simulink subsystem "rss_FaltResp"  (R2023a)
settings: Solver=VariableStepAuto  StartTime=0.0  StopTime=10.0  RelTol=1e-3
undefined symbols (not defined in the file): Cdbl_numFaltDiaNum, ENM_SYS_STATUS, Gbol_enLmpHmeStop_C, Gs16_nLmpHmeRefMechSpd_C, Gs16_nMaxRefMechSpd_C, Gs16_nMotoTmpStallRefMechSpd_C, Gs16_trqTmpStallTqUpLim_C, Gs16_trqTqUpLim_C, Gu16_ctLmpHmeDurCnt_C, Gu16_uLimHmeSplyVltgConfTrs_C, Gu16_uLimHmeSplyVltgRcvyTrs_C
libraries: simulink x5, vhit_control_library x1
settings Model: Creator=xiaoqiang.yuan  LastModifiedBy=xiaoqiang.yuan

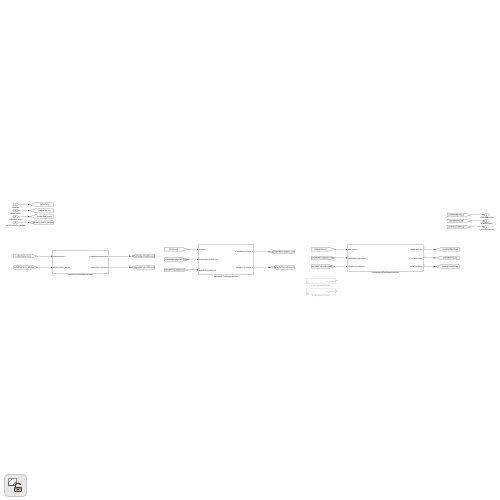
[thumbnail: Simulink's stored preview of the top-level diagram]
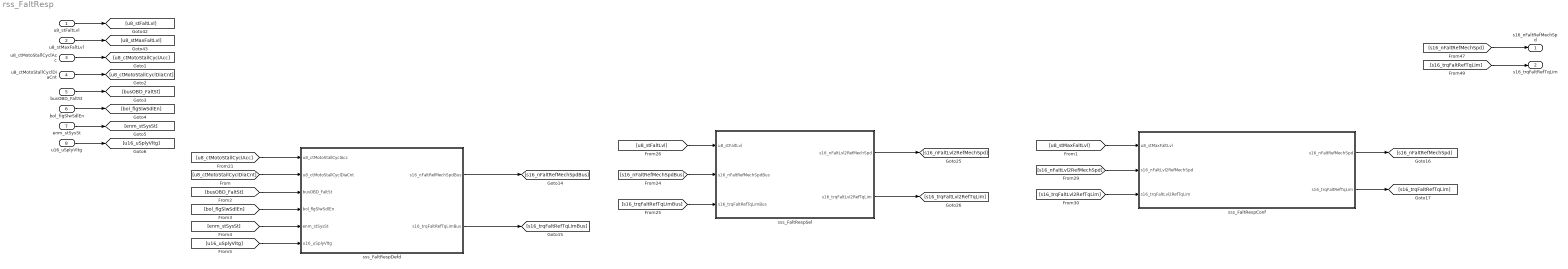
== system rss_FaltResp ==
  u8_stFaltLvl : Inport  OutDataTypeStr=uint8
  u8_stMaxFaltLvl : Inport  Port=2  OutDataTypeStr=uint8
  u8_ctMotoStallCyclAcc : Inport  Port=3  OutDataTypeStr=uint8
  u8_ctMotoStallCyclDiaCnt : Inport  Port=4  OutDataTypeStr=uint8
  busOBD_FaltSt : Inport  Port=5  OutDataTypeStr=Bus: BUS_OBD_FALT_STS
  bol_flgSlwSdlEn : Inport  Port=6  OutDataTypeStr=boolean
  enm_stSysSt : Inport  Port=7  OutDataTypeStr=Enum: ENM_SYS_STATUS
  u16_uSplyVltg : Inport  Port=8
  sss_FaltRespConf : Subsystem
  sss_FaltRespDefd : Subsystem
  sss_FaltRespSel : Subsystem
  s16_nFaltRefMechSpd : Outport  OutDataTypeStr=dt_Standardize_s16p15b0
  s16_trqFaltRefTqLim : Outport  Port=2  OutDataTypeStr=dt_Standardize_s16p15b0
  wires:
  u8_stFaltLvl/1 -> [u8_stFaltLvl]
  u8_stMaxFaltLvl/1 -> [u8_stMaxFaltLvl]
  u8_ctMotoStallCyclAcc/1 -> [u8_ctMotoStallCyclAcc]
  [u8_ctMotoStallCyclAcc] -> sss_FaltRespDefd/1(u8_ctMotoStallCyclAcc)
  sss_FaltRespDefd/1(s16_nFaltRefMechSpdBus) -> [s16_nFaltRefMechSpdBus]
  sss_FaltRespDefd/2(s16_trqFaltRefTqLimBus) -> [s16_trqFaltRefTqLimBus]
  [s16_trqFaltRefTqLimBus] -> sss_FaltRespSel/3(s16_trqFaltRefTqLimBus)
  [s16_nFaltRefMechSpdBus] -> sss_FaltRespSel/2(s16_nFaltRefMechSpdBus)
  [u8_stFaltLvl] -> sss_FaltRespSel/1(u8_stFaltLvl)
  sss_FaltRespSel/2(s16_trqFaltLvl2RefTqLim) -> [s16_trqFaltLvl2RefTqLim]
  sss_FaltRespSel/1(s16_nFaltLvl2RefMechSpd) -> [s16_nFaltLvl2RefMechSpd]
  sss_FaltRespConf/1(s16_nFaltRefMechSpd) -> [s16_nFaltRefMechSpd]
  sss_FaltRespConf/2(s16_trqFaltRefTqLim) -> [s16_trqFaltRefTqLim]
  [s16_nFaltRefMechSpd] -> s16_nFaltRefMechSpd/1
  [s16_trqFaltRefTqLim] -> s16_trqFaltRefTqLim/1
  [u8_stMaxFaltLvl] -> sss_FaltRespConf/1(u8_stMaxFaltLvl)
  u8_ctMotoStallCyclDiaCnt/1 -> [u8_ctMotoStallCyclDiaCnt]
  [u8_ctMotoStallCyclDiaCnt] -> sss_FaltRespDefd/2(u8_ctMotoStallCyclDiaCnt)
  busOBD_FaltSt/1 -> [busOBD_FaltSt]
  [busOBD_FaltSt] -> sss_FaltRespDefd/3(busOBD_FaltSt)
  bol_flgSlwSdlEn/1 -> [bol_flgSlwSdlEn]
  [bol_flgSlwSdlEn] -> sss_FaltRespDefd/4(bol_flgSlwSdlEn)
  enm_stSysSt/1 -> [enm_stSysSt]
  [enm_stSysSt] -> sss_FaltRespDefd/5(enm_stSysSt)
  [s16_nFaltLvl2RefMechSpd] -> sss_FaltRespConf/2(s16_nFaltLvl2RefMechSpd)
  [s16_trqFaltLvl2RefTqLim] -> sss_FaltRespConf/3(s16_trqFaltLvl2RefTqLim)
  u16_uSplyVltg/1 -> [u16_uSplyVltg]
  [u16_uSplyVltg] -> sss_FaltRespDefd/6(u16_uSplyVltg)

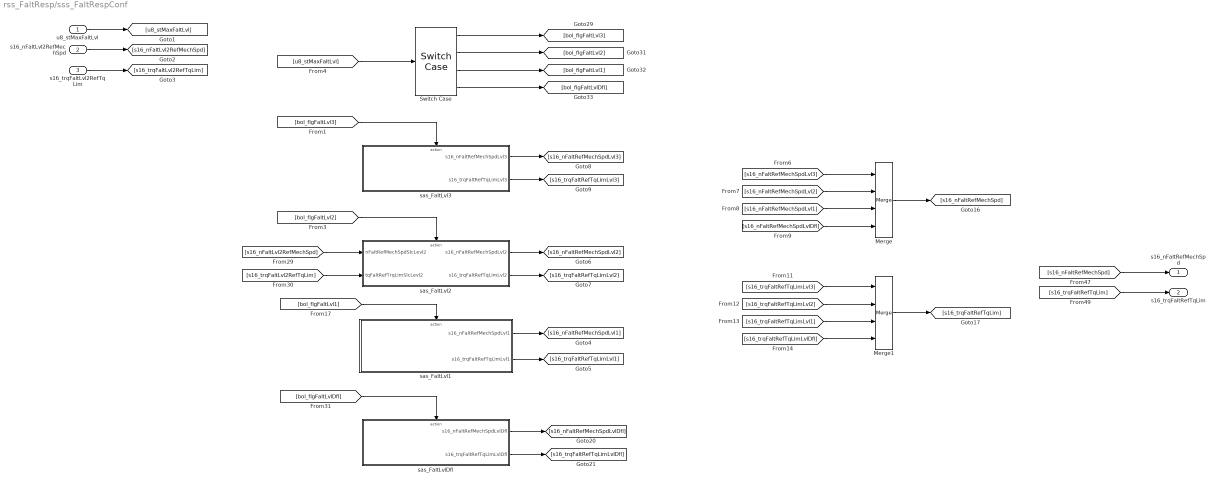
== system rss_FaltResp/sss_FaltRespConf ==
  u8_stMaxFaltLvl : Inport
  s16_nFaltLvl2RefMechSpd : Inport  Port=2
  s16_trqFaltLvl2RefTqLim : Inport  Port=3
  Merge : Merge  Inputs=4
  Merge1 : Merge  Inputs=4
  Switch Case : SwitchCase  CaseConditions={3,2,1}
  sas_FaltLvl1 : Subsystem  TreatAsAtomicUnit=on
  sas_FaltLvl2 : Subsystem  TreatAsAtomicUnit=on
  sas_FaltLvl3 : Subsystem  TreatAsAtomicUnit=on
  sas_FaltLvlDfl : Subsystem  TreatAsAtomicUnit=on
  s16_nFaltRefMechSpd : Outport
  s16_trqFaltRefTqLim : Outport  Port=2
  wires:
  [s16_trqFaltRefTqLimLvlDfl] -> Merge1/4
  [s16_trqFaltRefTqLimLvl1] -> Merge1/3
  [s16_trqFaltRefTqLimLvl2] -> Merge1/2
  [s16_trqFaltRefTqLimLvl3] -> Merge1/1
  [s16_nFaltRefMechSpdLvlDfl] -> Merge/4
  [s16_nFaltRefMechSpdLvl1] -> Merge/3
  [s16_nFaltRefMechSpdLvl2] -> Merge/2
  [s16_nFaltRefMechSpdLvl3] -> Merge/1
  Switch Case/2 -> [bol_flgFaltLvl2]
  s16_trqFaltLvl2RefTqLim/1 -> [s16_trqFaltLvl2RefTqLim]
  s16_nFaltLvl2RefMechSpd/1 -> [s16_nFaltLvl2RefMechSpd]
  u8_stMaxFaltLvl/1 -> [u8_stMaxFaltLvl]
  sas_FaltLvl1/1(s16_nFaltRefMechSpdLvl1) -> [s16_nFaltRefMechSpdLvl1]
  sas_FaltLvl1/2(s16_trqFaltRefTqLimLvl1) -> [s16_trqFaltRefTqLimLvl1]
  sas_FaltLvlDfl/1(s16_nFaltRefMechSpdLvlDfl) -> [s16_nFaltRefMechSpdLvlDfl]
  Merge/1 -> [s16_nFaltRefMechSpd]
  [s16_nFaltLvl2RefMechSpd] -> sas_FaltLvl2/1(nFaltRefMechSpdSlcLevl2)
  sas_FaltLvl3/1(s16_nFaltRefMechSpdLvl3) -> [s16_nFaltRefMechSpdLvl3]
  [bol_flgFaltLvlDfl] -> sas_FaltLvlDfl/Action
  sas_FaltLvl3/2(s16_trqFaltRefTqLimLvl3) -> [s16_trqFaltRefTqLimLvl3]
  sas_FaltLvlDfl/2(s16_trqFaltRefTqLimLvlDfl) -> [s16_trqFaltRefTqLimLvlDfl]
  [bol_flgFaltLvl2] -> sas_FaltLvl2/Action
  Switch Case/4 -> [bol_flgFaltLvlDfl]
  Merge1/1 -> [s16_trqFaltRefTqLim]
  Switch Case/3 -> [bol_flgFaltLvl1]
  [u8_stMaxFaltLvl] -> Switch Case/1
  [s16_trqFaltRefTqLim] -> s16_trqFaltRefTqLim/1
  [bol_flgFaltLvl3] -> sas_FaltLvl3/Action
  sas_FaltLvl2/2(s16_trqFaltRefTqLimLvl2) -> [s16_trqFaltRefTqLimLvl2]
  sas_FaltLvl2/1(s16_nFaltRefMechSpdLvl2) -> [s16_nFaltRefMechSpdLvl2]
  [bol_flgFaltLvl1] -> sas_FaltLvl1/Action
  Switch Case/1 -> [bol_flgFaltLvl3]
  [s16_trqFaltLvl2RefTqLim] -> sas_FaltLvl2/2(tqFaltRefTrqLimSlcLevl2)
  [s16_nFaltRefMechSpd] -> s16_nFaltRefMechSpd/1

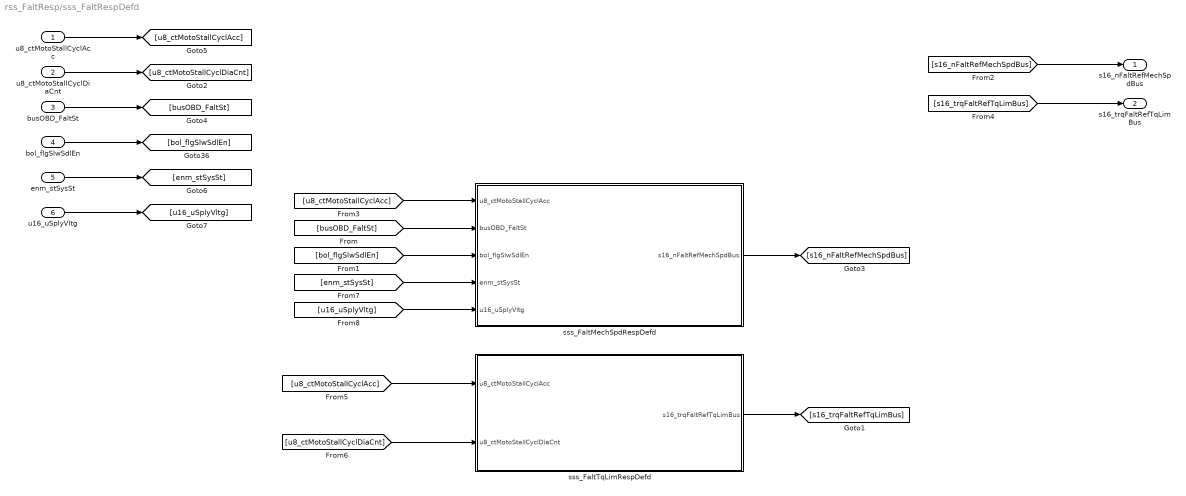
== system rss_FaltResp/sss_FaltRespDefd ==
  u8_ctMotoStallCyclAcc : Inport
  u8_ctMotoStallCyclDiaCnt : Inport  Port=2
  busOBD_FaltSt : Inport  Port=3
  bol_flgSlwSdlEn : Inport  Port=4
  enm_stSysSt : Inport  Port=5
  u16_uSplyVltg : Inport  Port=6
  sss_FaltMechSpdRespDefd : Subsystem
  sss_FaltTqLimRespDefd : Subsystem
  s16_nFaltRefMechSpdBus : Outport
  s16_trqFaltRefTqLimBus : Outport  Port=2
  wires:
  [u16_uSplyVltg] -> sss_FaltMechSpdRespDefd/5(u16_uSplyVltg)
  u16_uSplyVltg/1 -> [u16_uSplyVltg]
  [enm_stSysSt] -> sss_FaltMechSpdRespDefd/4(enm_stSysSt)
  enm_stSysSt/1 -> [enm_stSysSt]
  [bol_flgSlwSdlEn] -> sss_FaltMechSpdRespDefd/3(bol_flgSlwSdlEn)
  bol_flgSlwSdlEn/1 -> [bol_flgSlwSdlEn]
  [busOBD_FaltSt] -> sss_FaltMechSpdRespDefd/2(busOBD_FaltSt)
  busOBD_FaltSt/1 -> [busOBD_FaltSt]
  [u8_ctMotoStallCyclAcc] -> sss_FaltMechSpdRespDefd/1(u8_ctMotoStallCyclAcc)
  sss_FaltTqLimRespDefd/1(s16_trqFaltRefTqLimBus) -> [s16_trqFaltRefTqLimBus]
  sss_FaltMechSpdRespDefd/1(s16_nFaltRefMechSpdBus) -> [s16_nFaltRefMechSpdBus]
  [u8_ctMotoStallCyclDiaCnt] -> sss_FaltTqLimRespDefd/2(u8_ctMotoStallCyclDiaCnt)
  [u8_ctMotoStallCyclAcc] -> sss_FaltTqLimRespDefd/1(u8_ctMotoStallCyclAcc)
  u8_ctMotoStallCyclDiaCnt/1 -> [u8_ctMotoStallCyclDiaCnt]
  u8_ctMotoStallCyclAcc/1 -> [u8_ctMotoStallCyclAcc]
  [s16_trqFaltRefTqLimBus] -> s16_trqFaltRefTqLimBus/1
  [s16_nFaltRefMechSpdBus] -> s16_nFaltRefMechSpdBus/1

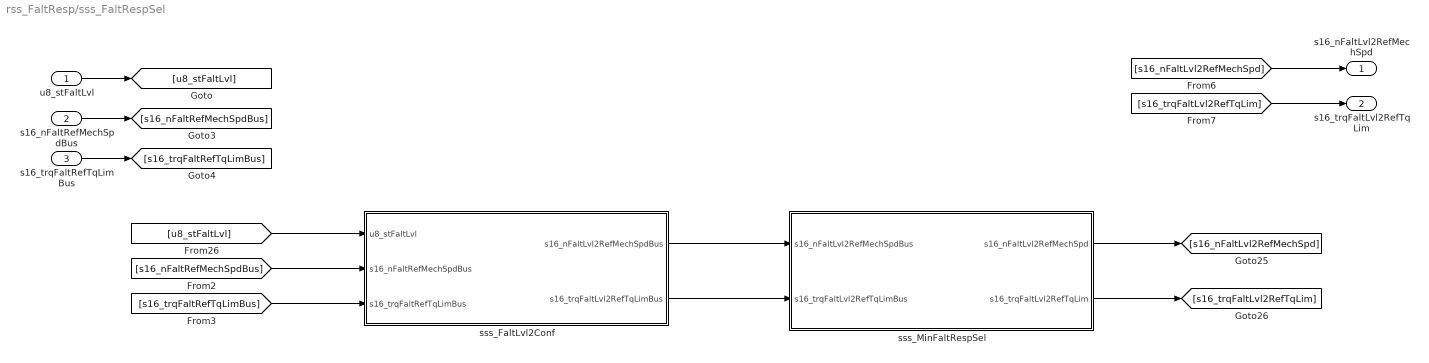
== system rss_FaltResp/sss_FaltRespSel ==
  u8_stFaltLvl : Inport
  s16_nFaltRefMechSpdBus : Inport  Port=2
  s16_trqFaltRefTqLimBus : Inport  Port=3
  sss_FaltLvl2Conf : Subsystem  TreatAsAtomicUnit=on
      settings: RTWSystemCode=Nonreusable function
  sss_MinFaltRespSel : Subsystem
      settings: RTWSystemCode=Nonreusable function
  s16_nFaltLvl2RefMechSpd : Outport
  s16_trqFaltLvl2RefTqLim : Outport  Port=2
  wires:
  sss_FaltLvl2Conf/2(s16_trqFaltLvl2RefTqLimBus) -> sss_MinFaltRespSel/2(s16_trqFaltLvl2RefTqLimBus)
  sss_FaltLvl2Conf/1(s16_nFaltLvl2RefMechSpdBus) -> sss_MinFaltRespSel/1(s16_nFaltLvl2RefMechSpdBus)
  sss_MinFaltRespSel/2(s16_trqFaltLvl2RefTqLim) -> [s16_trqFaltLvl2RefTqLim]
  sss_MinFaltRespSel/1(s16_nFaltLvl2RefMechSpd) -> [s16_nFaltLvl2RefMechSpd]
  [s16_trqFaltLvl2RefTqLim] -> s16_trqFaltLvl2RefTqLim/1
  [s16_nFaltLvl2RefMechSpd] -> s16_nFaltLvl2RefMechSpd/1
  [s16_trqFaltRefTqLimBus] -> sss_FaltLvl2Conf/3(s16_trqFaltRefTqLimBus)
  [s16_nFaltRefMechSpdBus] -> sss_FaltLvl2Conf/2(s16_nFaltRefMechSpdBus)
  [u8_stFaltLvl] -> sss_FaltLvl2Conf/1(u8_stFaltLvl)
  s16_nFaltRefMechSpdBus/1 -> [s16_nFaltRefMechSpdBus]
  s16_trqFaltRefTqLimBus/1 -> [s16_trqFaltRefTqLimBus]
  u8_stFaltLvl/1 -> [u8_stFaltLvl]

== system rss_FaltResp/sss_FaltRespConf/sas_FaltLvl1 ==
  Action Port : ActionPort
  Constant : Constant  Value=Gs16_nMaxRefMechSpd_C
  Constant1 : Constant  Value=Gs16_trqTqUpLim_C
  s16_nFaltRefMechSpdLvl1 : Outport
  s16_trqFaltRefTqLimLvl1 : Outport  Port=2
  wires:
  Constant/1 -> s16_nFaltRefMechSpdLvl1/1
  Constant1/1 -> s16_trqFaltRefTqLimLvl1/1

== system rss_FaltResp/sss_FaltRespConf/sas_FaltLvl2 ==
  nFaltRefMechSpdSlcLevl2 : Inport
  tqFaltRefTrqLimSlcLevl2 : Inport  Port=2
  Action Port : ActionPort
  s16_nFaltRefMechSpdLvl2 : Outport
  s16_trqFaltRefTqLimLvl2 : Outport  Port=2
  wires:
  nFaltRefMechSpdSlcLevl2/1 -> s16_nFaltRefMechSpdLvl2/1
  tqFaltRefTrqLimSlcLevl2/1 -> s16_trqFaltRefTqLimLvl2/1

== system rss_FaltResp/sss_FaltRespConf/sas_FaltLvl3 ==
  Action Port : ActionPort
  Constant : Constant  Value=0  OutDataTypeStr=dt_Standardize_s16p15b0
  Constant1 : Constant  Value=0  OutDataTypeStr=dt_Standardize_s16p15b0
  s16_nFaltRefMechSpdLvl3 : Outport
  s16_trqFaltRefTqLimLvl3 : Outport  Port=2
  wires:
  Constant/1 -> s16_nFaltRefMechSpdLvl3/1
  Constant1/1 -> s16_trqFaltRefTqLimLvl3/1

== system rss_FaltResp/sss_FaltRespConf/sas_FaltLvlDfl ==
  Action Port : ActionPort
  Constant : Constant  Value=Gs16_nMaxRefMechSpd_C
  Constant1 : Constant  Value=Gs16_trqTqUpLim_C
  s16_nFaltRefMechSpdLvlDfl : Outport
  s16_trqFaltRefTqLimLvlDfl : Outport  Port=2
  wires:
  Constant/1 -> s16_nFaltRefMechSpdLvlDfl/1
  Constant1/1 -> s16_trqFaltRefTqLimLvlDfl/1

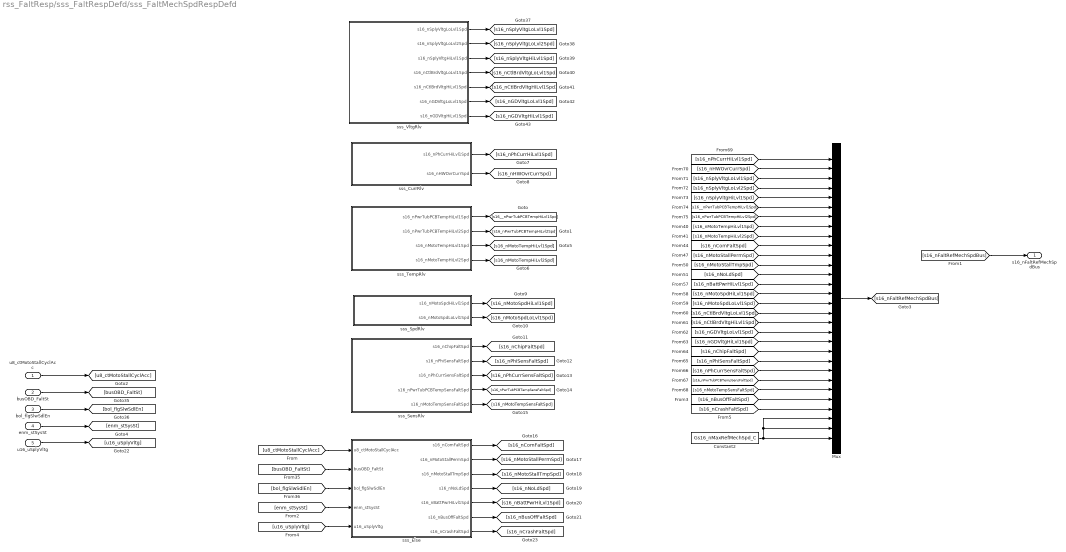
== system rss_FaltResp/sss_FaltRespDefd/sss_FaltMechSpdRespDefd ==
  u8_ctMotoStallCyclAcc : Inport
  busOBD_FaltSt : Inport  Port=2
  bol_flgSlwSdlEn : Inport  Port=3
  enm_stSysSt : Inport  Port=4
  u16_uSplyVltg : Inport  Port=5
  Constant2 : Constant  Value=Gs16_nMaxRefMechSpd_C
  Mux : Mux  Inputs=30
  sss_CurrRlv : Subsystem
  sss_Else : Subsystem
  sss_SensRlv : Subsystem
  sss_SpdRlv : Subsystem
  sss_TempRlv : Subsystem
  sss_VltgRlv : Subsystem
  s16_nFaltRefMechSpdBus : Outport
  wires:
  [s16_nCrashFaltSpd] -> Mux/27
  sss_Else/7(s16_nCrashFaltSpd) -> [s16_nCrashFaltSpd]
  [u16_uSplyVltg] -> sss_Else/5(u16_uSplyVltg)
  u16_uSplyVltg/1 -> [u16_uSplyVltg]
  [s16_nBusOffFaltSpd] -> Mux/26
  sss_Else/6(s16_nBusOffFaltSpd) -> [s16_nBusOffFaltSpd]
  [enm_stSysSt] -> sss_Else/4(enm_stSysSt)
  enm_stSysSt/1 -> [enm_stSysSt]
  [u8_ctMotoStallCyclAcc] -> sss_Else/1(u8_ctMotoStallCyclAcc)
  [bol_flgSlwSdlEn] -> sss_Else/3(bol_flgSlwSdlEn)
  [busOBD_FaltSt] -> sss_Else/2(busOBD_FaltSt)
  sss_Else/1(s16_nComFaltSpd) -> [s16_nComFaltSpd]
  sss_Else/2(s16_nMotoStallPermSpd) -> [s16_nMotoStallPermSpd]
  sss_Else/3(s16_nMotoStallTmpSpd) -> [s16_nMotoStallTmpSpd]
  sss_Else/4(s16_nNoLdSpd) -> [s16_nNoLdSpd]
  sss_Else/5(s16_nBattPwrHiLvl1Spd) -> [s16_nBattPwrHiLvl1Spd]
  sss_SensRlv/5(s16_nMotoTempSensFaltSpd) -> [s16_nMotoTempSensFaltSpd]
  sss_SensRlv/4(s16_nPwrTubPCBTempSensFaltSpd) -> [s16_nPwrTubPCBTempSensFaltSpd]
  sss_SensRlv/3(s16_nPhCurrSensFaltSpd) -> [s16_nPhCurrSensFaltSpd]
  sss_SensRlv/2(s16_nPhiSensFaltSpd) -> [s16_nPhiSensFaltSpd]
  sss_SensRlv/1(s16_nChipFaltSpd) -> [s16_nChipFaltSpd]
  sss_SpdRlv/2(s16_nMotoSpdLoLvl1Spd) -> [s16_nMotoSpdLoLvl1Spd]
  sss_SpdRlv/1(s16_nMotoSpdHiLvl1Spd) -> [s16_nMotoSpdHiLvl1Spd]
  sss_TempRlv/4(s16_nMotoTempHiLvl2Spd) -> [s16_nMotoTempHiLvl2Spd]
  sss_TempRlv/3(s16_nMotoTempHiLvl1Spd) -> [s16_nMotoTempHiLvl1Spd]
  sss_TempRlv/2(s16_nPwrTubPCBTempHiLvl2Spd) -> [s16_nPwrTubPCBTempHiLvl2Spd]
  sss_TempRlv/1(s16_nPwrTubPCBTempHiLvl1Spd) -> [s16__nPwrTubPCBTempHiLvl1Spd]
  sss_CurrRlv/2(s16_nHWOvrCurrSpd) -> [s16_nHWOvrCurrSpd]
  sss_CurrRlv/1(s16_nPhCurrHiLvl1Spd) -> [s16_nPhCurrHiLvl1Spd]
  Mux/1 -> [s16_nFaltRefMechSpdBus]
  [s16_nPhCurrSensFaltSpd] -> Mux/23
  [s16_nMotoStallTmpSpd] -> Mux/12
  Constant2/1 -> Mux/30, Mux/29, Mux/28
  [s16_nSplyVltgHiLvl1Spd] -> Mux/5
  [s16_nSplyVltgLoLvl1Spd] -> Mux/3
  [s16__nPwrTubPCBTempHiLvl1Spd] -> Mux/6
  [s16_nGDVltgLoLvl1Spd] -> Mux/19
  [s16_nHWOvrCurrSpd] -> Mux/2
  [s16_nMotoSpdHiLvl1Spd] -> Mux/15
  [s16_nPwrTubPCBTempSensFaltSpd] -> Mux/24
  [s16_nNoLdSpd] -> Mux/13
  [s16_nChipFaltSpd] -> Mux/21
  [s16_nMotoTempSensFaltSpd] -> Mux/25
  [s16_nPhCurrHiLvl1Spd] -> Mux/1
  [s16_nCtlBrdVltgLoLvl1Spd] -> Mux/17
  [s16_nPhiSensFaltSpd] -> Mux/22
  [s16_nGDVltgHiLvl1Spd] -> Mux/20
  [s16_nCtlBrdVltgHiLvl1Spd] -> Mux/18
  [s16_nComFaltSpd] -> Mux/10
  [s16_nMotoSpdLoLvl1Spd] -> Mux/16
  [s16_nMotoStallPermSpd] -> Mux/11
  [s16_nBattPwrHiLvl1Spd] -> Mux/14
  [s16_nPwrTubPCBTempHiLvl2Spd] -> Mux/7
  [s16_nMotoTempHiLvl1Spd] -> Mux/8
  [s16_nMotoTempHiLvl2Spd] -> Mux/9
  [s16_nSplyVltgLoLvl2Spd] -> Mux/4
  bol_flgSlwSdlEn/1 -> [bol_flgSlwSdlEn]
  busOBD_FaltSt/1 -> [busOBD_FaltSt]
  [s16_nFaltRefMechSpdBus] -> s16_nFaltRefMechSpdBus/1
  u8_ctMotoStallCyclAcc/1 -> [u8_ctMotoStallCyclAcc]
  sss_VltgRlv/5(s16_nCtlBrdVltgHiLvl1Spd) -> [s16_nCtlBrdVltgHiLvl1Spd]
  sss_VltgRlv/6(s16_nGDVltgLoLvl1Spd) -> [s16_nGDVltgLoLvl1Spd]
  sss_VltgRlv/2(s16_nSplyVltgLoLvl2Spd) -> [s16_nSplyVltgLoLvl2Spd]
  sss_VltgRlv/3(s16_nSplyVltgHiLvl1Spd) -> [s16_nSplyVltgHiLvl1Spd]
  sss_VltgRlv/7(s16_nGDVltgHiLvl1Spd) -> [s16_nGDVltgHiLvl1Spd]
  sss_VltgRlv/4(s16_nCtlBrdVltgLoLvl1Spd) -> [s16_nCtlBrdVltgLoLvl1Spd]
  sss_VltgRlv/1(s16_nSplyVltgLoLvl1Spd) -> [s16_nSplyVltgLoLvl1Spd]

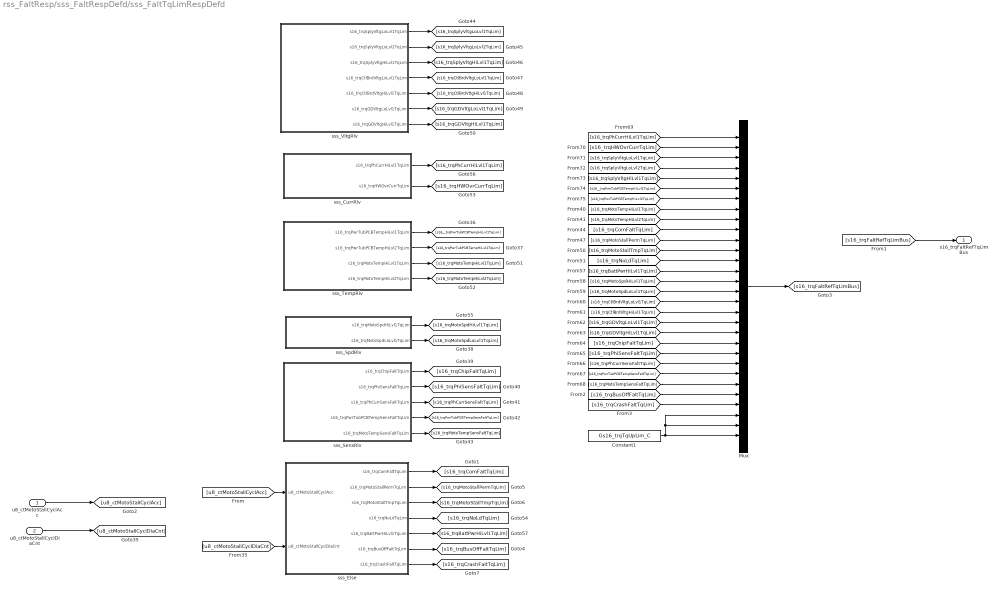
== system rss_FaltResp/sss_FaltRespDefd/sss_FaltTqLimRespDefd ==
  u8_ctMotoStallCyclAcc : Inport
  u8_ctMotoStallCyclDiaCnt : Inport  Port=2
  Constant1 : Constant  Value=Gs16_trqTqUpLim_C
  Mux : Mux  Inputs=30
  sss_CurrRlv : Subsystem
  sss_Else : Subsystem
  sss_SensRlv : Subsystem
  sss_SpdRlv : Subsystem
  sss_TempRlv : Subsystem
  sss_VltgRlv : Subsystem
  s16_trqFaltRefTqLimBus : Outport
  wires:
  [s16_trqCrashFaltTqLim] -> Mux/27
  sss_Else/7(s16_trqCrashFaltTqLim) -> [s16_trqCrashFaltTqLim]
  [s16_trqBusOffFaltTqLim] -> Mux/26
  sss_Else/6(s16_trqBusOffFaltTqLim) -> [s16_trqBusOffFaltTqLim]
  [u8_ctMotoStallCyclDiaCnt] -> sss_Else/2(u8_ctMotoStallCyclDiaCnt)
  [u8_ctMotoStallCyclAcc] -> sss_Else/1(u8_ctMotoStallCyclAcc)
  sss_Else/4(s16_trqNoLdTqLim) -> [s16_trqNoLdTqLim]
  sss_Else/3(s16_trqMotoStallTmpTqLim) -> [s16_trqMotoStallTmpTqLim]
  sss_Else/1(s16_trqComFaltTqLim) -> [s16_trqComFaltTqLim]
  sss_Else/2(s16_trqMotoStallPermTqLim) -> [s16_trqMotoStallPermTqLim]
  sss_Else/5(s16_trqBattPwrHiLvl1TqLim) -> [s16_trqBattPwrHiLvl1TqLim]
  sss_SensRlv/3(s16_trqPhCurrSensFaltTqLim) -> [s16_trqPhCurrSensFaltTqLim]
  sss_SpdRlv/1(s16_trqMotoSpdHiLvl1TqLim) -> [s16_trqMotoSpdHiLvl1TqLim]
  sss_TempRlv/3(s16_trqMotoTempHiLvl1TqLim) -> [s16_trqMotoTempHiLvl1TqLim]
  sss_TempRlv/1(s16_trqPwrTubPCBTempHiLvl1TqLim) -> [s16__trqPwrTubPCBTempHiLvl1TqLim]
  sss_VltgRlv/2(s16_trqSplyVltgLoLvl2TqLim) -> [s16_trqSplyVltgLoLvl2TqLim]
  sss_CurrRlv/2(s16_trqHWOvrCurrTqLim) -> [s16_trqHWOvrCurrTqLim]
  sss_SensRlv/1(s16_trqChipFaltTqLim) -> [s16_trqChipFaltTqLim]
  sss_SpdRlv/2(s16_trqMotoSpdLoLvl1TqLim) -> [s16_trqMotoSpdLoLvl1TqLim]
  sss_TempRlv/4(s16_trqMotoTempHiLvl2TqLim) -> [s16_trqMotoTempHiLvl2TqLim]
  sss_VltgRlv/6(s16_trqGDVltgLoLvl1TqLim) -> [s16_trqGDVltgLoLvl1TqLim]
  sss_VltgRlv/3(s16_trqSplyVltgHiLvl1TqLim) -> [s16_trqSplyVltgHiLvl1TqLim]
  sss_SensRlv/2(s16_trqPhiSensFaltTqLim) -> [s16_trqPhiSensFaltTqLim]
  sss_SensRlv/4(s16_trqPwrTubPCBTempSensFaltTqLim) -> [s16_trqPwrTubPCBTempSensFaltTqLim]
  sss_VltgRlv/5(s16_trqCtlBrdVltgHiLvl1TqLim) -> [s16_trqCtlBrdVltgHiLvl1TqLim]
  sss_SensRlv/5(s16_trqMotoTempSensFaltTqLim) -> [s16_trqMotoTempSensFaltTqLim]
  sss_TempRlv/2(s16_trqPwrTubPCBTempHiLvl2TqLim) -> [s16_trqPwrTubPCBTempHiLvl2TqLim]
  sss_CurrRlv/1(s16_trqPhCurrHiLvl1TqLim) -> [s16_trqPhCurrHiLvl1TqLim]
  sss_VltgRlv/1(s16_trqSplyVltgLoLvl1TqLim) -> [s16_trqSplyVltgLoLvl1TqLim]
  sss_VltgRlv/4(s16_trqCtlBrdVltgLoLvl1TqLim) -> [s16_trqCtlBrdVltgLoLvl1TqLim]
  sss_VltgRlv/7(s16_trqGDVltgHiLvl1TqLim) -> [s16_trqGDVltgHiLvl1TqLim]
  Mux/1 -> [s16_trqFaltRefTqLimBus]
  [s16_trqChipFaltTqLim] -> Mux/21
  [s16_trqMotoTempHiLvl1TqLim] -> Mux/8
  [s16_trqMotoStallTmpTqLim] -> Mux/12
  [s16_trqPwrTubPCBTempHiLvl2TqLim] -> Mux/7
  [s16_trqPhCurrSensFaltTqLim] -> Mux/23
  [s16_trqMotoTempHiLvl2TqLim] -> Mux/9
  [s16_trqSplyVltgLoLvl2TqLim] -> Mux/4
  [s16_trqMotoStallPermTqLim] -> Mux/11
  [s16_trqComFaltTqLim] -> Mux/10
  [s16_trqCtlBrdVltgLoLvl1TqLim] -> Mux/17
  [s16_trqBattPwrHiLvl1TqLim] -> Mux/14
  [s16_trqGDVltgHiLvl1TqLim] -> Mux/20
  [s16_trqPhCurrHiLvl1TqLim] -> Mux/1
  [s16_trqMotoTempSensFaltTqLim] -> Mux/25
  [s16_trqCtlBrdVltgHiLvl1TqLim] -> Mux/18
  [s16_trqPhiSensFaltTqLim] -> Mux/22
  [s16_trqMotoSpdLoLvl1TqLim] -> Mux/16
  [s16__trqPwrTubPCBTempHiLvl1TqLim] -> Mux/6
  [s16_trqHWOvrCurrTqLim] -> Mux/2
  [s16_trqNoLdTqLim] -> Mux/13
  [s16_trqGDVltgLoLvl1TqLim] -> Mux/19
  [s16_trqMotoSpdHiLvl1TqLim] -> Mux/15
  [s16_trqSplyVltgLoLvl1TqLim] -> Mux/3
  [s16_trqSplyVltgHiLvl1TqLim] -> Mux/5
  [s16_trqPwrTubPCBTempSensFaltTqLim] -> Mux/24
  Constant1/1 -> Mux/30, Mux/29, Mux/28
  u8_ctMotoStallCyclDiaCnt/1 -> [u8_ctMotoStallCyclDiaCnt]
  u8_ctMotoStallCyclAcc/1 -> [u8_ctMotoStallCyclAcc]
  [s16_trqFaltRefTqLimBus] -> s16_trqFaltRefTqLimBus/1

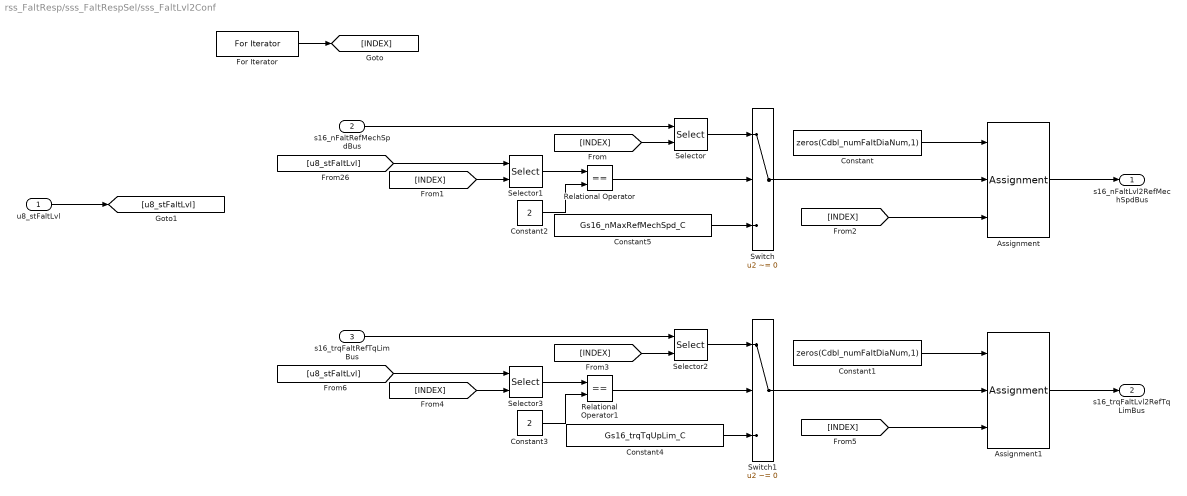
== system rss_FaltResp/sss_FaltRespSel/sss_FaltLvl2Conf ==
  u8_stFaltLvl : Inport
  s16_nFaltRefMechSpdBus : Inport  Port=2
  s16_trqFaltRefTqLimBus : Inport  Port=3
  Assignment : Assignment  DiagnosticForDimensions=Warning  IndexOptions=Index vector (port)  Indices=1  OutputSizes=1
  Assignment1 : Assignment  DiagnosticForDimensions=Warning  IndexOptions=Index vector (port)  Indices=1  OutputSizes=1
  Constant : Constant  Value=zeros(Cdbl_numFaltDiaNum,1)  OutDataTypeStr=dt_Standardize_s16p15b0
  Constant1 : Constant  Value=zeros(Cdbl_numFaltDiaNum,1)  OutDataTypeStr=dt_Standardize_s16p15b0
  Constant2 : Constant  Value=2  OutDataTypeStr=uint8
  Constant3 : Constant  Value=2  OutDataTypeStr=uint8
  Constant4 : Constant  Value=Gs16_trqTqUpLim_C
  Constant5 : Constant  Value=Gs16_nMaxRefMechSpd_C
  For Iterator : ForIterator  IterationLimit=Cdbl_numFaltDiaNum  IterationVariableDataType=uint8
  Relational Operator : RelationalOperator  Operator===  OutDataTypeStr=boolean  RndMeth=Simplest  InputSameDT=off
  Relational Operator1 : RelationalOperator  Operator===  OutDataTypeStr=boolean  RndMeth=Simplest  InputSameDT=off
  Selector{,1..3} (4 alike) : Selector  InputPortWidth=Cdbl_numFaltDiaNum  IndexOptions=Index vector (port)  Indices=[1 3]  OutputSizes=1
  Switch : Switch  Criteria=u2 ~= 0  SaturateOnIntegerOverflow=off  InputSameDT=off
  Switch1 : Switch  Criteria=u2 ~= 0  SaturateOnIntegerOverflow=off  InputSameDT=off
  s16_nFaltLvl2RefMechSpdBus : Outport
  s16_trqFaltLvl2RefTqLimBus : Outport  Port=2
  wires:
  [INDEX] -> Assignment/3
  Constant/1 -> Assignment/1
  Switch/1 -> Assignment/2
  [INDEX] -> Selector1/2
  [INDEX] -> Selector/2
  For Iterator/1 -> [INDEX]
  s16_nFaltRefMechSpdBus/1 -> Selector/1
  Constant5/1 -> Switch/3
  Selector/1 -> Switch/1
  Selector1/1 -> Relational Operator/1
  Constant2/1 -> Relational Operator/2
  Relational Operator/1 -> Switch/2
  Assignment/1 -> s16_nFaltLvl2RefMechSpdBus/1
  u8_stFaltLvl/1 -> [u8_stFaltLvl]
  [u8_stFaltLvl] -> Selector1/1
  Relational Operator1/1 -> Switch1/2
  [u8_stFaltLvl] -> Selector3/1
  Assignment1/1 -> s16_trqFaltLvl2RefTqLimBus/1
  Constant3/1 -> Relational Operator1/2
  Selector2/1 -> Switch1/1
  [INDEX] -> Assignment1/3
  Switch1/1 -> Assignment1/2
  [INDEX] -> Selector2/2
  Constant1/1 -> Assignment1/1
  [INDEX] -> Selector3/2
  Selector3/1 -> Relational Operator1/1
  s16_trqFaltRefTqLimBus/1 -> Selector2/1
  Constant4/1 -> Switch1/3

== system rss_FaltResp/sss_FaltRespSel/sss_MinFaltRespSel ==
  s16_nFaltLvl2RefMechSpdBus : Inport
  s16_trqFaltLvl2RefTqLimBus : Inport  Port=2
  Min : MinMax
  Min1 : MinMax
  s16_nFaltLvl2RefMechSpd : Outport
  s16_trqFaltLvl2RefTqLim : Outport  Port=2
  wires:
  s16_trqFaltLvl2RefTqLimBus/1 -> Min1/1
  Min1/1 -> s16_trqFaltLvl2RefTqLim/1
  Min/1 -> s16_nFaltLvl2RefMechSpd/1
  s16_nFaltLvl2RefMechSpdBus/1 -> Min/1

== system rss_FaltResp/sss_FaltRespDefd/sss_FaltMechSpdRespDefd/sss_CurrRlv ==
  Constant17 : Constant  Value=Gs16_nMaxRefMechSpd_C
  s16_nPhCurrHiLvl1Spd : Outport
  s16_nHWOvrCurrSpd : Outport  Port=2
  wires:
  Constant17/1 -> s16_nPhCurrHiLvl1Spd/1, s16_nHWOvrCurrSpd/1

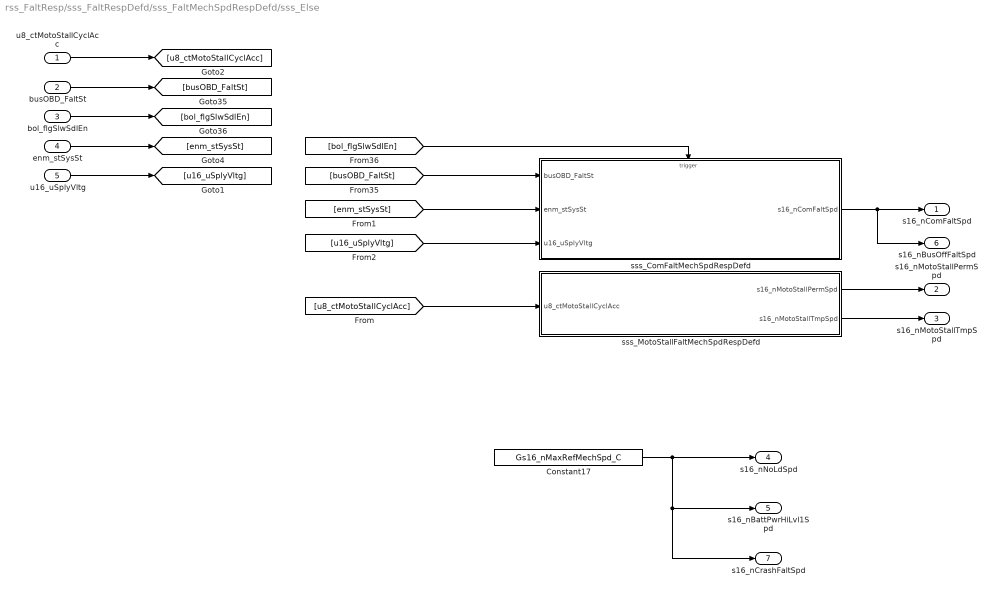
== system rss_FaltResp/sss_FaltRespDefd/sss_FaltMechSpdRespDefd/sss_Else ==
  u8_ctMotoStallCyclAcc : Inport
  busOBD_FaltSt : Inport  Port=2
  bol_flgSlwSdlEn : Inport  Port=3
  enm_stSysSt : Inport  Port=4
  u16_uSplyVltg : Inport  Port=5
  Constant17 : Constant  Value=Gs16_nMaxRefMechSpd_C
  sss_ComFaltMechSpdRespDefd : Subsystem  Variant=on  VariantControlMode=label  VariantControl=Choice  LabelModeActiveChoice=GEELY_PROJECT
  sss_MotoStallFaltMechSpdRespDefd : Subsystem
  s16_nComFaltSpd : Outport
  s16_nMotoStallPermSpd : Outport  Port=2
  s16_nMotoStallTmpSpd : Outport  Port=3
  s16_nNoLdSpd : Outport  Port=4
  s16_nBattPwrHiLvl1Spd : Outport  Port=5
  s16_nBusOffFaltSpd : Outport  Port=6
  s16_nCrashFaltSpd : Outport  Port=7
  wires:
  [u16_uSplyVltg] -> sss_ComFaltMechSpdRespDefd/3(u16_uSplyVltg)
  u16_uSplyVltg/1 -> [u16_uSplyVltg]
  sss_ComFaltMechSpdRespDefd/1(s16_nComFaltSpd) -> s16_nComFaltSpd/1, s16_nBusOffFaltSpd/1
  [bol_flgSlwSdlEn] -> sss_ComFaltMechSpdRespDefd/Trigger
  [enm_stSysSt] -> sss_ComFaltMechSpdRespDefd/2(enm_stSysSt)
  [busOBD_FaltSt] -> sss_ComFaltMechSpdRespDefd/1(busOBD_FaltSt)
  enm_stSysSt/1 -> [enm_stSysSt]
  Constant17/1 -> s16_nNoLdSpd/1, s16_nBattPwrHiLvl1Spd/1, s16_nCrashFaltSpd/1
  u8_ctMotoStallCyclAcc/1 -> [u8_ctMotoStallCyclAcc]
  busOBD_FaltSt/1 -> [busOBD_FaltSt]
  bol_flgSlwSdlEn/1 -> [bol_flgSlwSdlEn]
  [u8_ctMotoStallCyclAcc] -> sss_MotoStallFaltMechSpdRespDefd/1(u8_ctMotoStallCyclAcc)
  sss_MotoStallFaltMechSpdRespDefd/2(s16_nMotoStallTmpSpd) -> s16_nMotoStallTmpSpd/1
  sss_MotoStallFaltMechSpdRespDefd/1(s16_nMotoStallPermSpd) -> s16_nMotoStallPermSpd/1

== system rss_FaltResp/sss_FaltRespDefd/sss_FaltMechSpdRespDefd/sss_SensRlv ==
  Constant17 : Constant  Value=Gs16_nMaxRefMechSpd_C
  s16_nChipFaltSpd : Outport
  s16_nPhiSensFaltSpd : Outport  Port=2
  s16_nPhCurrSensFaltSpd : Outport  Port=3
  s16_nPwrTubPCBTempSensFaltSpd : Outport  Port=4
  s16_nMotoTempSensFaltSpd : Outport  Port=5
  wires:
  Constant17/1 -> s16_nChipFaltSpd/1, s16_nPhiSensFaltSpd/1, s16_nPhCurrSensFaltSpd/1, s16_nPwrTubPCBTempSensFaltSpd/1, s16_nMotoTempSensFaltSpd/1

== system rss_FaltResp/sss_FaltRespDefd/sss_FaltMechSpdRespDefd/sss_SpdRlv ==
  Constant17 : Constant  Value=Gs16_nMaxRefMechSpd_C
  s16_nMotoSpdHiLvl1Spd : Outport
  s16_nMotoSpdLoLvl1Spd : Outport  Port=2
  wires:
  Constant17/1 -> s16_nMotoSpdHiLvl1Spd/1, s16_nMotoSpdLoLvl1Spd/1

== system rss_FaltResp/sss_FaltRespDefd/sss_FaltMechSpdRespDefd/sss_TempRlv ==
  Constant17 : Constant  Value=Gs16_nMaxRefMechSpd_C
  s16_nPwrTubPCBTempHiLvl1Spd : Outport
  s16_nPwrTubPCBTempHiLvl2Spd : Outport  Port=2
  s16_nMotoTempHiLvl1Spd : Outport  Port=3
  s16_nMotoTempHiLvl2Spd : Outport  Port=4
  wires:
  Constant17/1 -> s16_nPwrTubPCBTempHiLvl1Spd/1, s16_nPwrTubPCBTempHiLvl2Spd/1, s16_nMotoTempHiLvl1Spd/1, s16_nMotoTempHiLvl2Spd/1

== system rss_FaltResp/sss_FaltRespDefd/sss_FaltMechSpdRespDefd/sss_VltgRlv ==
  Constant17 : Constant  Value=Gs16_nMaxRefMechSpd_C
  s16_nSplyVltgLoLvl1Spd : Outport
  s16_nSplyVltgLoLvl2Spd : Outport  Port=2
  s16_nSplyVltgHiLvl1Spd : Outport  Port=3
  s16_nCtlBrdVltgLoLvl1Spd : Outport  Port=4
  s16_nCtlBrdVltgHiLvl1Spd : Outport  Port=5
  s16_nGDVltgLoLvl1Spd : Outport  Port=6
  s16_nGDVltgHiLvl1Spd : Outport  Port=7
  wires:
  Constant17/1 -> s16_nSplyVltgLoLvl1Spd/1, s16_nSplyVltgLoLvl2Spd/1, s16_nSplyVltgHiLvl1Spd/1, s16_nCtlBrdVltgLoLvl1Spd/1, s16_nCtlBrdVltgHiLvl1Spd/1, s16_nGDVltgLoLvl1Spd/1, s16_nGDVltgHiLvl1Spd/1

== system rss_FaltResp/sss_FaltRespDefd/sss_FaltTqLimRespDefd/sss_CurrRlv ==
  Constant1 : Constant  Value=Gs16_trqTqUpLim_C
  s16_trqPhCurrHiLvl1TqLim : Outport
  s16_trqHWOvrCurrTqLim : Outport  Port=2
  wires:
  Constant1/1 -> s16_trqPhCurrHiLvl1TqLim/1, s16_trqHWOvrCurrTqLim/1

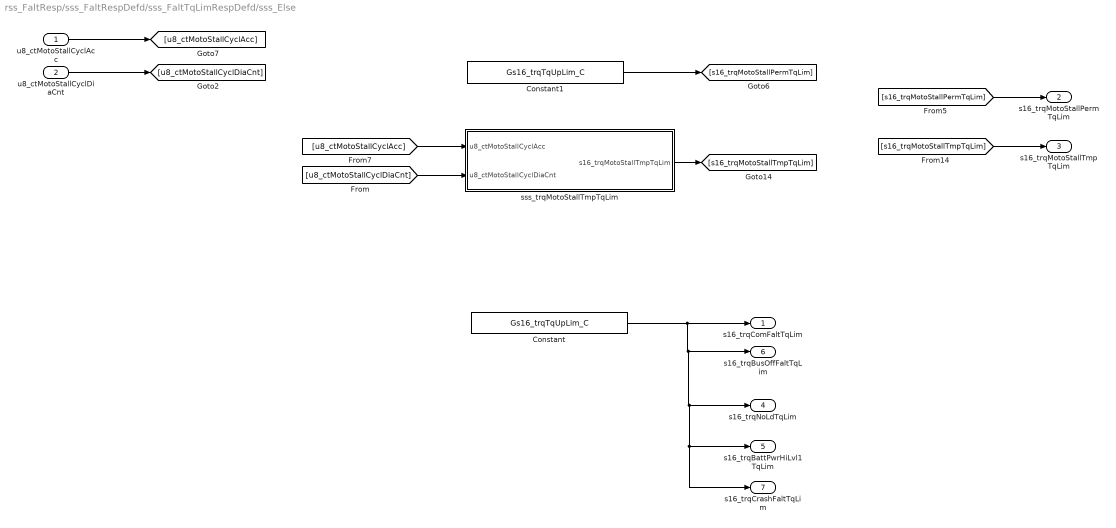
== system rss_FaltResp/sss_FaltRespDefd/sss_FaltTqLimRespDefd/sss_Else ==
  u8_ctMotoStallCyclAcc : Inport
  u8_ctMotoStallCyclDiaCnt : Inport  Port=2
  Constant : Constant  Value=Gs16_trqTqUpLim_C
  Constant1 : Constant  Value=Gs16_trqTqUpLim_C
  sss_trqMotoStallTmpTqLim : Subsystem
  s16_trqComFaltTqLim : Outport
  s16_trqMotoStallPermTqLim : Outport  Port=2
  s16_trqMotoStallTmpTqLim : Outport  Port=3
  s16_trqNoLdTqLim : Outport  Port=4
  s16_trqBattPwrHiLvl1TqLim : Outport  Port=5
  s16_trqBusOffFaltTqLim : Outport  Port=6
  s16_trqCrashFaltTqLim : Outport  Port=7
  wires:
  [s16_trqMotoStallPermTqLim] -> s16_trqMotoStallPermTqLim/1
  [u8_ctMotoStallCyclAcc] -> sss_trqMotoStallTmpTqLim/1(u8_ctMotoStallCyclAcc)
  [u8_ctMotoStallCyclDiaCnt] -> sss_trqMotoStallTmpTqLim/2(u8_ctMotoStallCyclDiaCnt)
  u8_ctMotoStallCyclAcc/1 -> [u8_ctMotoStallCyclAcc]
  [s16_trqMotoStallTmpTqLim] -> s16_trqMotoStallTmpTqLim/1
  Constant1/1 -> [s16_trqMotoStallPermTqLim]
  sss_trqMotoStallTmpTqLim/1(s16_trqMotoStallTmpTqLim) -> [s16_trqMotoStallTmpTqLim]
  u8_ctMotoStallCyclDiaCnt/1 -> [u8_ctMotoStallCyclDiaCnt]
  Constant/1 -> s16_trqComFaltTqLim/1, s16_trqBusOffFaltTqLim/1, s16_trqNoLdTqLim/1, s16_trqBattPwrHiLvl1TqLim/1, s16_trqCrashFaltTqLim/1

== system rss_FaltResp/sss_FaltRespDefd/sss_FaltTqLimRespDefd/sss_SensRlv ==
  Constant1 : Constant  Value=Gs16_trqTqUpLim_C
  s16_trqChipFaltTqLim : Outport
  s16_trqPhiSensFaltTqLim : Outport  Port=2
  s16_trqPhCurrSensFaltTqLim : Outport  Port=3
  s16_trqPwrTubPCBTempSensFaltTqLim : Outport  Port=4
  s16_trqMotoTempSensFaltTqLim : Outport  Port=5
  wires:
  Constant1/1 -> s16_trqChipFaltTqLim/1, s16_trqPhiSensFaltTqLim/1, s16_trqPhCurrSensFaltTqLim/1, s16_trqPwrTubPCBTempSensFaltTqLim/1, s16_trqMotoTempSensFaltTqLim/1

== system rss_FaltResp/sss_FaltRespDefd/sss_FaltTqLimRespDefd/sss_SpdRlv ==
  Constant1 : Constant  Value=Gs16_trqTqUpLim_C
  s16_trqMotoSpdHiLvl1TqLim : Outport
  s16_trqMotoSpdLoLvl1TqLim : Outport  Port=2
  wires:
  Constant1/1 -> s16_trqMotoSpdHiLvl1TqLim/1, s16_trqMotoSpdLoLvl1TqLim/1

== system rss_FaltResp/sss_FaltRespDefd/sss_FaltTqLimRespDefd/sss_TempRlv ==
  Constant1 : Constant  Value=Gs16_trqTqUpLim_C
  s16_trqPwrTubPCBTempHiLvl1TqLim : Outport
  s16_trqPwrTubPCBTempHiLvl2TqLim : Outport  Port=2
  s16_trqMotoTempHiLvl1TqLim : Outport  Port=3
  s16_trqMotoTempHiLvl2TqLim : Outport  Port=4
  wires:
  Constant1/1 -> s16_trqPwrTubPCBTempHiLvl1TqLim/1, s16_trqPwrTubPCBTempHiLvl2TqLim/1, s16_trqMotoTempHiLvl1TqLim/1, s16_trqMotoTempHiLvl2TqLim/1

== system rss_FaltResp/sss_FaltRespDefd/sss_FaltTqLimRespDefd/sss_VltgRlv ==
  Constant1 : Constant  Value=Gs16_trqTqUpLim_C
  s16_trqSplyVltgLoLvl1TqLim : Outport
  s16_trqSplyVltgLoLvl2TqLim : Outport  Port=2
  s16_trqSplyVltgHiLvl1TqLim : Outport  Port=3
  s16_trqCtlBrdVltgLoLvl1TqLim : Outport  Port=4
  s16_trqCtlBrdVltgHiLvl1TqLim : Outport  Port=5
  s16_trqGDVltgLoLvl1TqLim : Outport  Port=6
  s16_trqGDVltgHiLvl1TqLim : Outport  Port=7
  wires:
  Constant1/1 -> s16_trqSplyVltgLoLvl1TqLim/1, s16_trqSplyVltgLoLvl2TqLim/1, s16_trqSplyVltgHiLvl1TqLim/1, s16_trqCtlBrdVltgLoLvl1TqLim/1, s16_trqCtlBrdVltgHiLvl1TqLim/1, s16_trqGDVltgLoLvl1TqLim/1, s16_trqGDVltgHiLvl1TqLim/1

== system rss_FaltResp/sss_FaltRespDefd/sss_FaltMechSpdRespDefd/sss_Else/sss_ComFaltMechSpdRespDefd ==
  busOBD_FaltSt : Inport
  enm_stSysSt : Inport  Port=2
  u16_uSplyVltg : Inport  Port=3
  Trigger : TriggerPort  VariantControl=(inherit)
  sss_ComFaltMechSpdRespDefd_CRRC : Subsystem  VariantControl=CRRC_PROJECT
  sss_ComFaltMechSpdRespDefd_GEELY : Subsystem  VariantControl=GEELY_PROJECT
  s16_nComFaltSpd : Outport

== system rss_FaltResp/sss_FaltRespDefd/sss_FaltMechSpdRespDefd/sss_Else/sss_MotoStallFaltMechSpdRespDefd ==
  u8_ctMotoStallCyclAcc : Inport
  Constant17 : Constant  Value=Gs16_nMaxRefMechSpd_C
  sss_MotoStallTmpSpd : Subsystem
  s16_nMotoStallPermSpd : Outport
  s16_nMotoStallTmpSpd : Outport  Port=2
  wires:
  Constant17/1 -> [s16_nMotoStallPermSpd]
  sss_MotoStallTmpSpd/1(s16_nMotoStallTmpSpd) -> [s16_nMotoStallTmpSpd]
  [u8_ctMotoStallCyclAcc] -> sss_MotoStallTmpSpd/1(u8_ctMotoStallCyclAcc)
  [s16_nMotoStallTmpSpd] -> s16_nMotoStallTmpSpd/1
  u8_ctMotoStallCyclAcc/1 -> [u8_ctMotoStallCyclAcc]
  [s16_nMotoStallPermSpd] -> s16_nMotoStallPermSpd/1

== system rss_FaltResp/sss_FaltRespDefd/sss_FaltTqLimRespDefd/sss_Else/sss_trqMotoStallTmpTqLim ==
  u8_ctMotoStallCyclAcc : Inport
  u8_ctMotoStallCyclDiaCnt : Inport  Port=2
  Constant1 : Constant  Value=Gs16_trqTmpStallTqUpLim_C
  Terminator : Terminator
  Terminator1 : Terminator
  s16_trqMotoStallTmpTqLim : Outport
  wires:
  u8_ctMotoStallCyclDiaCnt/1 -> Terminator1/1
  Constant1/1 -> s16_trqMotoStallTmpTqLim/1
  u8_ctMotoStallCyclAcc/1 -> Terminator/1

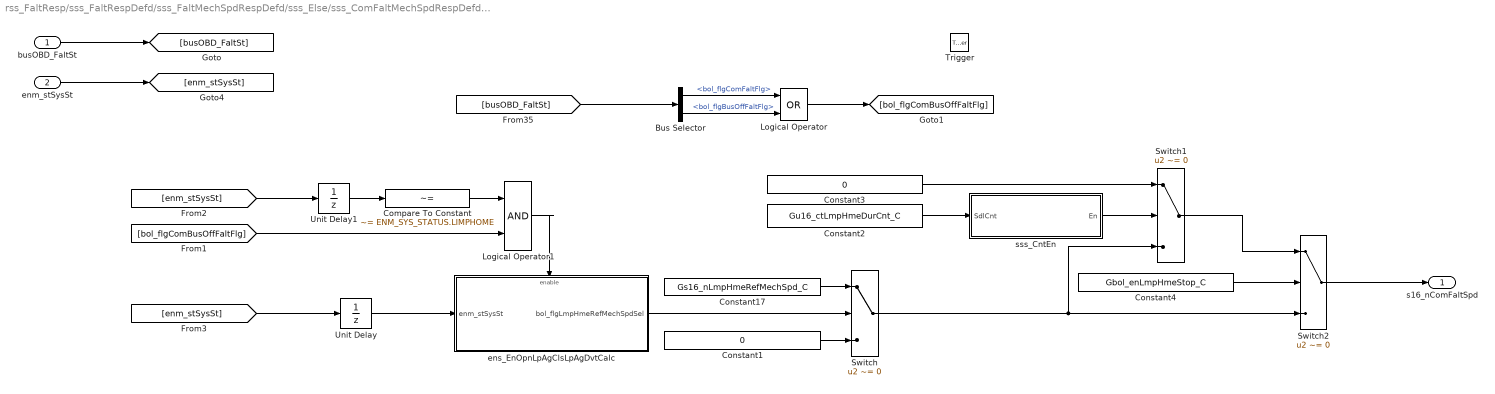
== system rss_FaltResp/sss_FaltRespDefd/sss_FaltMechSpdRespDefd/sss_Else/sss_ComFaltMechSpdRespDefd/sss_ComFaltMechSpdRespDefd_CRRC ==
  busOBD_FaltSt : Inport
  enm_stSysSt : Inport  Port=2
  Trigger : TriggerPort  VariantControl=(inherit)  PortDimensions=1
  Bus Selector : BusSelector  OutputSignals=bol_flgComFaltFlg,bol_flgBusOffFaltFlg
  Compare To Constant : simulink/Logic and Bit Operations/Compare To Constant  relop=~=  const=ENM_SYS_STATUS.LIMPHOME  OutDataTypeStr=boolean
  Constant1 : Constant  Value=0  OutDataTypeStr=dt_Standardize_s16p15b0
  Constant17 : Constant  Value=Gs16_nLmpHmeRefMechSpd_C
  Constant2 : Constant  Value=Gu16_ctLmpHmeDurCnt_C
  Constant3 : Constant  Value=0  OutDataTypeStr=dt_Standardize_s16p15b0
  Constant4 : Constant  Value=Gbol_enLmpHmeStop_C
  Logical Operator : Logic  Operator=OR  AllPortsSameDT=off  OutDataTypeStr=boolean
  Logical Operator1 : Logic  AllPortsSameDT=off  OutDataTypeStr=boolean
  Switch : Switch  Criteria=u2 ~= 0  SaturateOnIntegerOverflow=off  InputSameDT=off
  Switch1 : Switch  Criteria=u2 ~= 0  SaturateOnIntegerOverflow=off  InputSameDT=off
  Switch2 : Switch  Criteria=u2 ~= 0  SaturateOnIntegerOverflow=off  InputSameDT=off
  Unit Delay : UnitDelay  InitialCondition=ENM_SYS_STATUS.SYSINIT  SampleTime=-1  HasFrameUpgradeWarning=on
  Unit Delay1 : UnitDelay  InitialCondition=ENM_SYS_STATUS.SYSINIT  SampleTime=-1  HasFrameUpgradeWarning=on
  ens_EnOpnLpAgClsLpAgDvtCalc : Subsystem
  sss_CntEn : Subsystem  RTWFcnName=counter_10  RTWFileName=MotorControlLib
      settings: RTWFcnNameOpts=User specified  RTWFileNameOpts=User specified
  s16_nComFaltSpd : Outport
  wires:
  Switch2/1 -> s16_nComFaltSpd/1
  Switch1/1 -> Switch2/1
  Switch/1 -> Switch2/3, Switch1/3
  Constant4/1 -> Switch2/2
  Constant3/1 -> Switch1/1
  sss_CntEn/1(En) -> Switch1/2
  Constant2/1 -> sss_CntEn/1(SdlCnt)
  Unit Delay1/1 -> Compare To Constant/1
  [enm_stSysSt] -> Unit Delay1/1
  Unit Delay/1 -> ens_EnOpnLpAgClsLpAgDvtCalc/1(enm_stSysSt)
  Constant1/1 -> Switch/3
  Constant17/1 -> Switch/1
  ens_EnOpnLpAgClsLpAgDvtCalc/1(bol_flgLmpHmeRefMechSpdSel) -> Switch/2
  Compare To Constant/1 -> Logical Operator1/1
  enm_stSysSt/1 -> [enm_stSysSt]
  Logical Operator1/1 -> ens_EnOpnLpAgClsLpAgDvtCalc/Enable
  [bol_flgComBusOffFaltFlg] -> Logical Operator1/2
  Logical Operator/1 -> [bol_flgComBusOffFaltFlg]
  Bus Selector/1 -> Logical Operator/1  "<bol_flgComFaltFlg>"
  Bus Selector/2 -> Logical Operator/2  "<bol_flgBusOffFaltFlg>"
  [enm_stSysSt] -> Unit Delay/1
  [busOBD_FaltSt] -> Bus Selector/1
  busOBD_FaltSt/1 -> [busOBD_FaltSt]

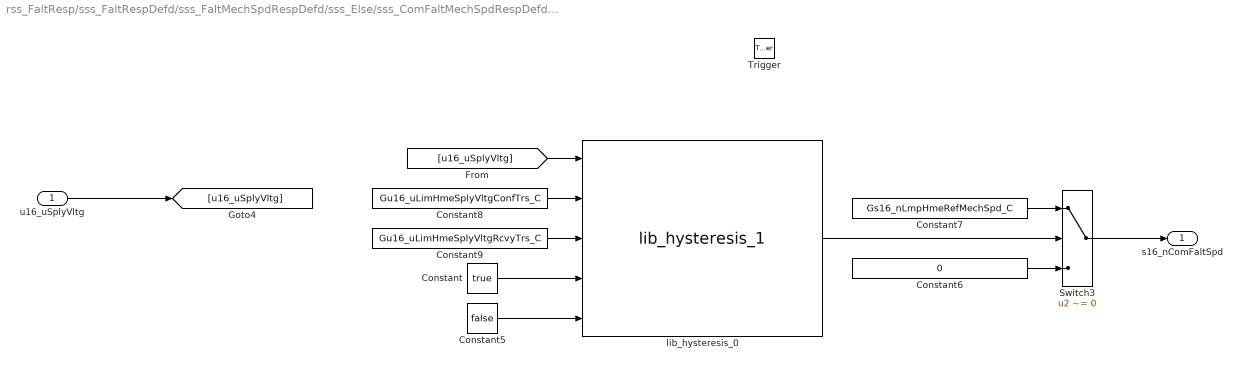
== system rss_FaltResp/sss_FaltRespDefd/sss_FaltMechSpdRespDefd/sss_Else/sss_ComFaltMechSpdRespDefd/sss_ComFaltMechSpdRespDefd_GEELY ==
  u16_uSplyVltg : Inport
  Trigger : TriggerPort  VariantControl=(inherit)  PortDimensions=1
  Constant : Constant  Value=true
  Constant5 : Constant  Value=false
  Constant6 : Constant  Value=0  OutDataTypeStr=dt_Standardize_s16p15b0
  Constant7 : Constant  Value=Gs16_nLmpHmeRefMechSpd_C
  Constant8 : Constant  Value=Gu16_uLimHmeSplyVltgConfTrs_C
  Constant9 : Constant  Value=Gu16_uLimHmeSplyVltgRcvyTrs_C
  Switch3 : Switch  Criteria=u2 ~= 0  SaturateOnIntegerOverflow=off  InputSameDT=off
  lib_hysteresis_0 : vhit_control_library/lib_hysteresis_1  lb_parInitOutp=1
  s16_nComFaltSpd : Outport
  wires:
  [u16_uSplyVltg] -> lib_hysteresis_0/1
  Constant9/1 -> lib_hysteresis_0/3
  Constant8/1 -> lib_hysteresis_0/2
  Switch3/1 -> s16_nComFaltSpd/1
  Constant6/1 -> Switch3/3
  Constant7/1 -> Switch3/1
  lib_hysteresis_0/1 -> Switch3/2
  Constant5/1 -> lib_hysteresis_0/5
  Constant/1 -> lib_hysteresis_0/4
  u16_uSplyVltg/1 -> [u16_uSplyVltg]

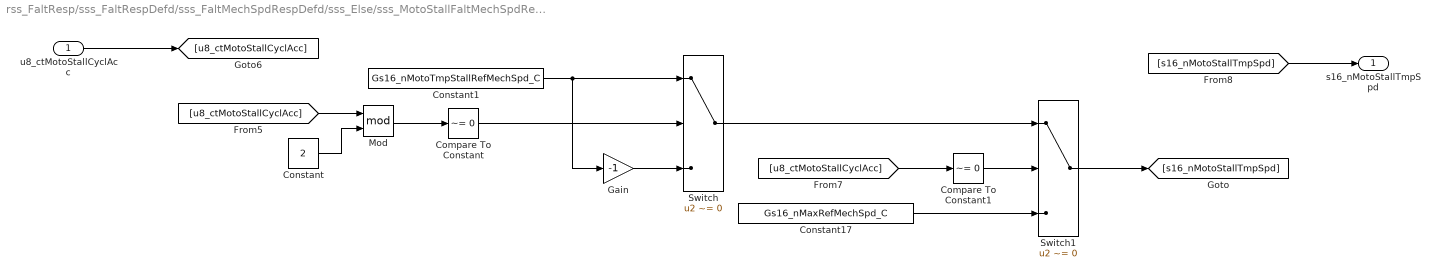
== system rss_FaltResp/sss_FaltRespDefd/sss_FaltMechSpdRespDefd/sss_Else/sss_MotoStallFaltMechSpdRespDefd/sss_MotoStallTmpSpd ==
  u8_ctMotoStallCyclAcc : Inport
  Compare To Constant : simulink/Logic and Bit Operations/Compare To Constant  relop=~=  const=0  OutDataTypeStr=boolean
  Compare To Constant1 : simulink/Logic and Bit Operations/Compare To Constant  relop=~=  const=0  OutDataTypeStr=boolean
  Constant : Constant  Value=2  OutDataTypeStr=uint8
  Constant1 : Constant  Value=Gs16_nMotoTmpStallRefMechSpd_C
  Constant17 : Constant  Value=Gs16_nMaxRefMechSpd_C
  Gain : Gain  Gain=-1  OutDataTypeStr=Inherit: Same as input
  Mod : Math  Operator=mod
  Switch : Switch  Criteria=u2 ~= 0  SaturateOnIntegerOverflow=off  InputSameDT=off
  Switch1 : Switch  Criteria=u2 ~= 0  SaturateOnIntegerOverflow=off  InputSameDT=off
  s16_nMotoStallTmpSpd : Outport
  wires:
  Constant1/1 -> Switch/1, Gain/1
  Gain/1 -> Switch/3
  Switch1/1 -> [s16_nMotoStallTmpSpd]
  [s16_nMotoStallTmpSpd] -> s16_nMotoStallTmpSpd/1
  Constant17/1 -> Switch1/3
  Compare To Constant1/1 -> Switch1/2
  [u8_ctMotoStallCyclAcc] -> Compare To Constant1/1
  [u8_ctMotoStallCyclAcc] -> Mod/1
  u8_ctMotoStallCyclAcc/1 -> [u8_ctMotoStallCyclAcc]
  Switch/1 -> Switch1/1
  Compare To Constant/1 -> Switch/2
  Mod/1 -> Compare To Constant/1
  Constant/1 -> Mod/2

== system rss_FaltResp/sss_FaltRespDefd/sss_FaltMechSpdRespDefd/sss_Else/sss_ComFaltMechSpdRespDefd/sss_ComFaltMechSpdRespDefd_CRRC/ens_EnOpnLpAgClsLpAgDvtCalc ==
  enm_stSysSt : Inport
  Enable : EnablePort
  Compare To Constant : simulink/Logic and Bit Operations/Compare To Constant  relop===  const=ENM_SYS_STATUS.RUN  OutDataTypeStr=boolean
  Compare To Constant1 : simulink/Logic and Bit Operations/Compare To Constant  relop===  const=ENM_SYS_STATUS.SYSDERATING  OutDataTypeStr=boolean
  Logical Operator2 : Logic  Operator=OR  AllPortsSameDT=off  OutDataTypeStr=boolean
  bol_flgLmpHmeRefMechSpdSel : Outport
  wires:
  Compare To Constant1/1 -> Logical Operator2/1
  enm_stSysSt/1 -> Compare To Constant1/1, Compare To Constant/1
  Compare To Constant/1 -> Logical Operator2/2
  Logical Operator2/1 -> bol_flgLmpHmeRefMechSpdSel/1

== system rss_FaltResp/sss_FaltRespDefd/sss_FaltMechSpdRespDefd/sss_Else/sss_ComFaltMechSpdRespDefd/sss_ComFaltMechSpdRespDefd_CRRC/sss_CntEn ==
  SdlCnt : Inport
      settings: AttributesFormatString=%<Description>cnt_max=n-1 n为总次数
  Add1 : Sum  OutDataTypeStr=Inherit: Same as first input
  Equal : RelationalOperator  Operator===  OutDataTypeStr=boolean
  Parameter2 : Constant  OutDataTypeStr=uint16  SampleTime=-1
      settings: AttributesFormatString=SampleTime=%<SampleTime>
  Switch : Switch  Criteria=u2 ~= 0  SaturateOnIntegerOverflow=off  OutDataTypeStr=Inherit: Same as first input
      settings: AttributesFormatString=InputSameDT=%<InputSameDT>
  Unit Delay : UnitDelay  InitialCondition=1  SampleTime=-1  HasFrameUpgradeWarning=on
  En : Outport
  wires:
  Add1/1 -> Switch/3
  Switch/1 -> Unit Delay/1
  Unit Delay/1 -> Equal/2, Add1/2, Switch/1
  Equal/1 -> En/1, Switch/2
  Parameter2/1 -> Add1/1
  SdlCnt/1 -> Equal/1
